simulink model "Exp ed2"  (R2016a)
settings: Solver=VariableStepAuto  StartTime=0.0  StopTime=10.0  RelTol=1e-3
settings Model: Creator=PAPUN  LastModifiedBy=PAPUN

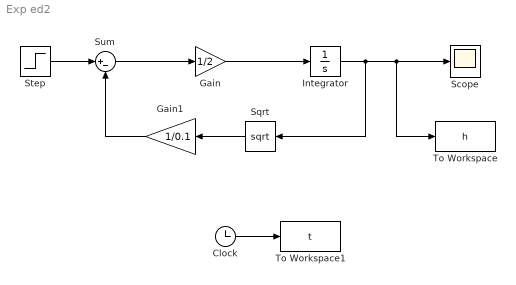
== system Exp ed2 ==
  Clock : Clock
  Gain : Gain  Gain=1/2
  Gain1 : Gain  Gain=1/0.1
  Integrator : Integrator
  Scope : Scope
  Sqrt : Sqrt  SaturateOnIntegerOverflow=on
  Step : Step  Time=0  SampleTime=0
  Sum : Sum  Inputs=|+-
  To Workspace : ToWorkspace  VariableName=h  SaveFormat=Timeseries  SampleTime=-1
  To Workspace1 : ToWorkspace  VariableName=t  SaveFormat=Timeseries  SampleTime=-1
  wires:
  Step/1 -> Sum/1
  Sum/1 -> Gain/1
  Gain/1 -> Integrator/1
  Integrator/1 -> Sqrt/1, To Workspace/1, Scope/1
  Sqrt/1 -> Gain1/1
  Gain1/1 -> Sum/2
  Clock/1 -> To Workspace1/1
